simulink model "while_iterator_subsystem"  (R2014a)
settings: Solver=FixedStepDiscrete  StartTime=0.0  StopTime=10.0  FixedStep=0.1  RelTol=1e-3
settings Model: BufferReuse=off  Creator=yoshi12  LastModifiedBy=ts1413
settings OptimizationCC: BlockReduction=off  OptimizeBlockIOStorage=off  BufferReuse=off  GlobalBufferReuse=off  ExpressionFolding=off  LocalBlockOutputs=off  OptimizeModelRefInitCode=on  LifeSpan=1
settings RTWCC: SystemTargetFile=ert.tlc  GenCodeOnly=on  TemplateMakefile=ert_default_tmf  Description=Embedded Coder  ProcessScript=ert_make_rtw_hook
settings CodeAppCC: IgnoreCustomStorageClasses=off
settings ERTTargetCC: ParMdlRefBuildCompliant=on  CompOptLevelCompliant=on  ConcurrentExecutionCompliant=on  ERTFirstTimeCompliant=on  ModelStepFunctionPrototypeControlCompliant=on  CPPClassGenCompliant=on  InlinedParameterPlacement=Hierarchical  ERTCustomFileTemplate=example_file_process.tlc

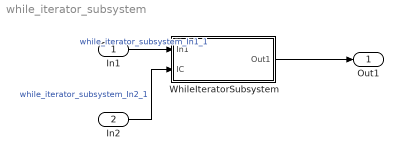
== system while_iterator_subsystem ==
  In1 : Inport
  In2 : Inport  Port=2
  WhileIteratorSubsystem : Subsystem  TreatAsAtomicUnit=on
  Out1 : Outport
  wires:
  In1/1 -> WhileIteratorSubsystem/1(In1)  "while_iterator_subsystem_In1_1"
  In2/1 -> WhileIteratorSubsystem/2(IC)  "while_iterator_subsystem_In2_1"
  WhileIteratorSubsystem/1(Out1) -> Out1/1

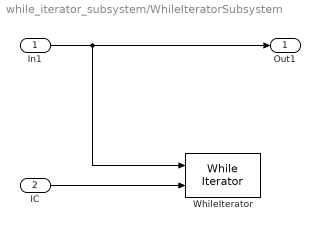
== system while_iterator_subsystem/WhileIteratorSubsystem ==
  In1 : Inport
  IC : Inport  Port=2
  WhileIterator : WhileIterator
  Out1 : Outport
  wires:
  IC/1 -> WhileIterator/2
  In1/1 -> WhileIterator/1, Out1/1
